simulink model "valve_02_sim"  (R2017b)
settings: Solver=VariableStepAuto  StartTime=0.0  StopTime=5  RelTol=1e-3
values from neighbouring files (symbols this model uses):
  fluid = nh3_v4    [valve_02.m]
undefined symbols (not defined in the file or in its folder): cp, cv, P, rho, T, Valve_regime, valveLib
libraries: simulink x4, thermochemical x4
settings Model: Creator=fferrucc  LastModifiedBy=fferrucc

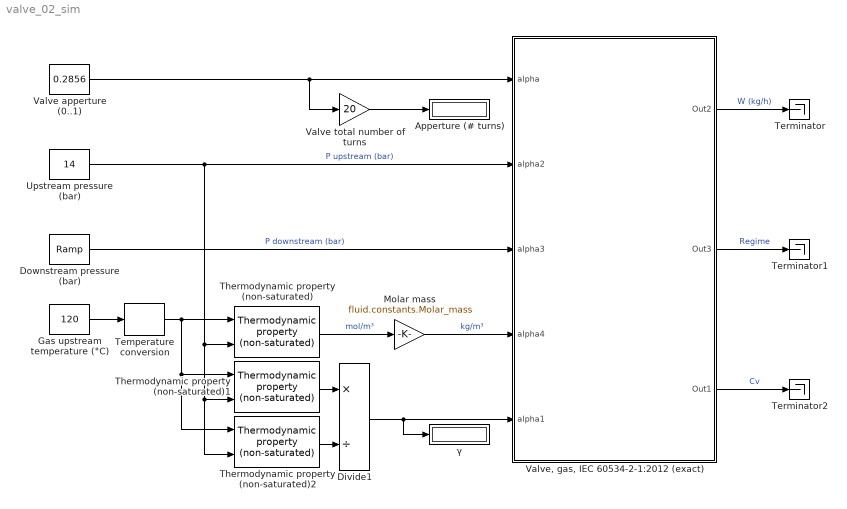
== system valve_02_sim ==
  Apperture (# turns) : Display
  Divide1 : Product  Inputs=*/
  "Downstream pressure (bar) " : simulink/Sources/Ramp  slope=1  start=0  X0=6
  Gas upstream temperature (°C) : Constant  Value=120
  Molar mass : Gain  Gain=fluid.constants.Molar_mass
  Temperature conversion : thermochemical/Conversions/Temperature conversion  sel=°C --> K
      settings: SourceProductName=@ Thermochemical
  Terminator : Terminator
  Terminator1 : Terminator
  Terminator2 : Terminator
  Thermodynamic property (non-saturated) : thermochemical/Thermodynamic fluid properties/Thermodynamic  property (non-saturated)  sel=rho(T,P)  fluid=fluid  reciprocVar=-1  lookup2D_BreakPoint1=fluid.no_sat.T_P_indep.var_indep.T  lookup2D_BreakPoint2=fluid.no_sat.T_P_indep.var_indep.P  lookup2D_Data=fluid.no_sat.T_P_indep.var_dep.rho_molar
      settings: SourceProductName=@ Thermochemical
  Thermodynamic property (non-saturated)1 : thermochemical/Thermodynamic fluid properties/Thermodynamic  property (non-saturated)  sel=cp(T,P)  fluid=fluid  reciprocVar=-1  lookup2D_BreakPoint1=fluid.no_sat.T_P_indep.var_indep.T  lookup2D_BreakPoint2=fluid.no_sat.T_P_indep.var_indep.P  lookup2D_Data=fluid.no_sat.T_P_indep.var_dep.Cp_molar
      settings: SourceProductName=@ Thermochemical
  Thermodynamic property (non-saturated)2 : thermochemical/Thermodynamic fluid properties/Thermodynamic  property (non-saturated)  sel=cv(T,P)  fluid=fluid  reciprocVar=-1  lookup2D_BreakPoint1=fluid.no_sat.T_P_indep.var_indep.T  lookup2D_BreakPoint2=fluid.no_sat.T_P_indep.var_indep.P  lookup2D_Data=fluid.no_sat.T_P_indep.var_dep.Cv_molar
      settings: SourceProductName=@ Thermochemical
  Upstream pressure (bar) : Constant  Value=14
  Valve apperture (0..1) : Constant  Value=0.2856
  Valve total number of turns : Gain  Gain=20
  "Valve, gas, IEC 60534-2-1:2012 (exact)" : Subsystem  AncestorBlock=thermochemical/Valves/Valve, gas, IEC 60534-2-1:2012 (exact)  mask(valve_gas_IEC60534_2_1_exact){Cv_dataPoints=valveLib.Hoke.s2300.model_2335G4Y.Cv_vs_apperture(:,2), apperture_dataPoints=valveLib.Hoke.s2300.model_2335G4Y.Cv_vs_apperture(:,1), xT=0.5}
      mask prompts: Cv_dataPoints "Cv vs apperture: Cv data points [0..Cv max]"; apperture_dataPoints "Cv vs apperture: apperture data points [0..1]"; xT "Pressure difference ratio factor of valve without attached fittings at choked flow ('xT' parameter) (use 0.5 if unknown)"
      mask help:
      | Model of a gas flow rate through a valve.
      |
      | The model takes into account the subcritical (non-chocked) and supercritical (chocked) regime of the pressure drop in the valve, switching its behaviour accordingly.
      |
      | The valve apperture is modulated by the signal 'apperture' (apperture = [0..1]).
      |
      | The model expects a table with the values of Cv (flow coeficient) as a function of the valve apperture (0..1).
      | NOTE: the relationship between Cv (imperial units) and Kv (SI units) is: Kv = 0.865*Cv.
      |
      | All the numerical outputs of the model are eigher positive or zero.
      mask DialogControl Control3 Prompt: Visit SWAGELOK site for more information about valves.
      mask DialogControl Control3 Callback: web('https://www.swagelok.com/en/Resources/CVCalculator','-browser')
  γ : Display
  wires:
  "Valve, gas, IEC 60534-2-1:2012 (exact)"/3(Out1) -> Terminator2/1  "Cv"
  "Valve, gas, IEC 60534-2-1:2012 (exact)"/2(Out3) -> Terminator1/1  "Regime"
  "Valve, gas, IEC 60534-2-1:2012 (exact)"/1(Out2) -> Terminator/1  "W (kg/h)"
  Thermodynamic property (non-saturated)/1 -> Molar mass/1  "mol/m³"
  Thermodynamic property (non-saturated)2/1 -> Divide1/2
  Thermodynamic property (non-saturated)1/1 -> Divide1/1
  Molar mass/1 -> "Valve, gas, IEC 60534-2-1:2012 (exact)"/4(alpha4)  "kg/m³"
  Upstream pressure (bar)/1 -> "Valve, gas, IEC 60534-2-1:2012 (exact)"/2(alpha2), Thermodynamic property (non-saturated)/2, Thermodynamic property (non-saturated)2/2, Thermodynamic property (non-saturated)1/2  "P upstream (bar)"
  Gas upstream temperature (°C)/1 -> Temperature conversion/1
  Divide1/1 -> γ/1, "Valve, gas, IEC 60534-2-1:2012 (exact)"/5(alpha1)
  Temperature conversion/1 -> Thermodynamic property (non-saturated)/1, Thermodynamic property (non-saturated)2/1, Thermodynamic property (non-saturated)1/1
  Valve apperture (0..1)/1 -> "Valve, gas, IEC 60534-2-1:2012 (exact)"/1(alpha), Valve total number of turns/1
  Valve total number of turns/1 -> Apperture (# turns)/1
  "Downstream pressure (bar) "/1 -> "Valve, gas, IEC 60534-2-1:2012 (exact)"/3(alpha3)  "P downstream (bar)"

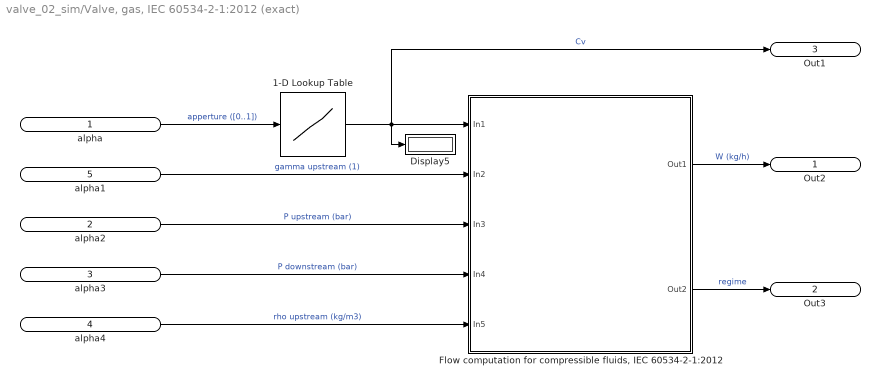
== system valve_02_sim/Valve, gas, IEC 60534-2-1:2012 (exact) ==
  alpha : Inport
  alpha2 : Inport  Port=2
  alpha3 : Inport  Port=3
  alpha4 : Inport  Port=4
  alpha1 : Inport  Port=5
  1-D Lookup Table : Lookup_n-D  NumberOfTableDimensions=1  BreakpointsForDimension1=apperture_dataPoints  BeginIndexSearchUsingPreviousIndexResult=on  Table=Cv_dataPoints  ExtrapMethod=Clip  InternalRulePriority=Speed  RndMeth=Simplest  InputSameDT=on
  Display5 : Display
  "Flow computation for compressible fluids, IEC 60534-2-1:2012" : Subsystem  LoadFcn=|
      | % For the 'regime' output to work, the model defines an enumerated type:
      | Simulink.defineIntEnumType('Valve_regime',{'Open_NonChocked','Closed','Open_Chocked'},[1 0 -1])
  Out2 : Outport
  Out3 : Outport  Port=2
  Out1 : Outport  Port=3
  wires:
  alpha4/1 -> "Flow computation for compressible fluids, IEC 60534-2-1:2012"/5(In5)  "rho upstream (kg/m3)"
  alpha3/1 -> "Flow computation for compressible fluids, IEC 60534-2-1:2012"/4(In4)  "P downstream (bar)"
  alpha2/1 -> "Flow computation for compressible fluids, IEC 60534-2-1:2012"/3(In3)  "P upstream (bar)"
  alpha1/1 -> "Flow computation for compressible fluids, IEC 60534-2-1:2012"/2(In2)  "gamma upstream (1)"
  1-D Lookup Table/1 -> "Flow computation for compressible fluids, IEC 60534-2-1:2012"/1(In1), Display5/1, Out1/1  "Cv"
  "Flow computation for compressible fluids, IEC 60534-2-1:2012"/2(Out2) -> Out3/1  "regime"
  alpha/1 -> 1-D Lookup Table/1  "apperture ([0..1])"
  "Flow computation for compressible fluids, IEC 60534-2-1:2012"/1(Out1) -> Out2/1  "W (kg/h)"

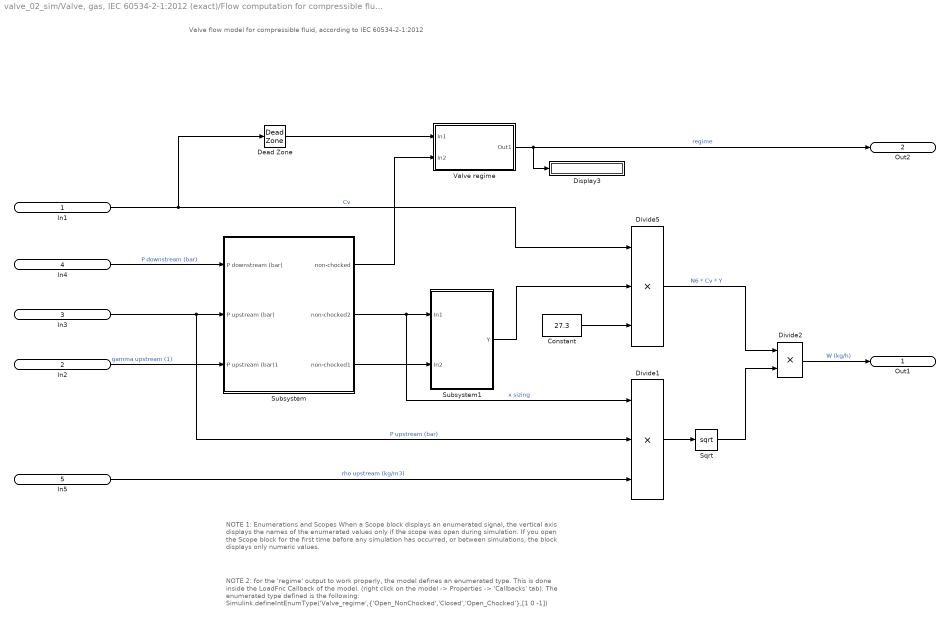
== system valve_02_sim/Valve, gas, IEC 60534-2-1:2012 (exact)/Flow computation for compressible fluids, IEC 60534-2-1:2012 ==
  note: NOTE 1: Enumerations and Scopes
      | When a Scope block displays an enumerated signal, the vertical axis displays the names of
      | the enumerated values only if the scope was open during simulation. If you open the Scope
      | block for the first time before any simulation has occurred, or between simulations, the block
      | displays only numeric values.
  note: NOTE 2: for the 'regime' output to work properly, the model defines an enumerated type. This is done
      | inside the LoadFnc Callback of the model. (right click on the model -> Properties -> 'Callbacks' tab).
      | The enumerated type defined is the following:
      | Simulink.defineIntEnumType('Valve_regime',{'Open_NonChocked','Closed','Open_Chocked'},[1 0 -1])
  note: Valve flow model for compressible fluid,
      | according to IEC 60534-2-1:2012
  In1 : Inport
  In2 : Inport  Port=2
  In3 : Inport  Port=3
  In4 : Inport  Port=4
  In5 : Inport  Port=5
  Constant : Constant  Value=27.3
  Dead Zone : DeadZone  LowerValue=-Inf  UpperValue=1e-7  SaturateOnIntegerOverflow=on
  Display3 : Display
  Divide1 : Product  Inputs=***
  Divide2 : Product  Inputs=**
  Divide5 : Product  Inputs=***
  Sqrt : Sqrt  SaturateOnIntegerOverflow=on
  Subsystem : Subsystem
  Subsystem1 : Subsystem
  Valve regime : Subsystem
  Out1 : Outport
  Out2 : Outport  Port=2
  wires:
  Dead Zone/1 -> Valve regime/1(In1)
  Valve regime/1(Out1) -> Display3/1, Out2/1  "regime"
  In4/1 -> Subsystem/1(P downstream (bar))  "P downstream (bar)"
  In3/1 -> Divide1/2, Subsystem/2(P upstream (bar))  "P upstream (bar)"
  In2/1 -> Subsystem/3(P upstream (bar)1)  "gamma upstream (1)"
  Subsystem/2(non-chocked2) -> Subsystem1/1(In1), Divide1/1  "x sizing"
  Subsystem/3(non-chocked1) -> Subsystem1/2(In2)
  In1/1 -> Dead Zone/1, Divide5/1  "Cv"
  Subsystem1/1(Y) -> Divide5/2
  Constant/1 -> Divide5/3
  Divide5/1 -> Divide2/1  "N6 * Cv * Y"
  In5/1 -> Divide1/3  "rho upstream (kg/m3)"
  Divide1/1 -> Sqrt/1
  Sqrt/1 -> Divide2/2
  Divide2/1 -> Out1/1  "W (kg/h)"
  Subsystem/1(non-chocked) -> Valve regime/2(In2)

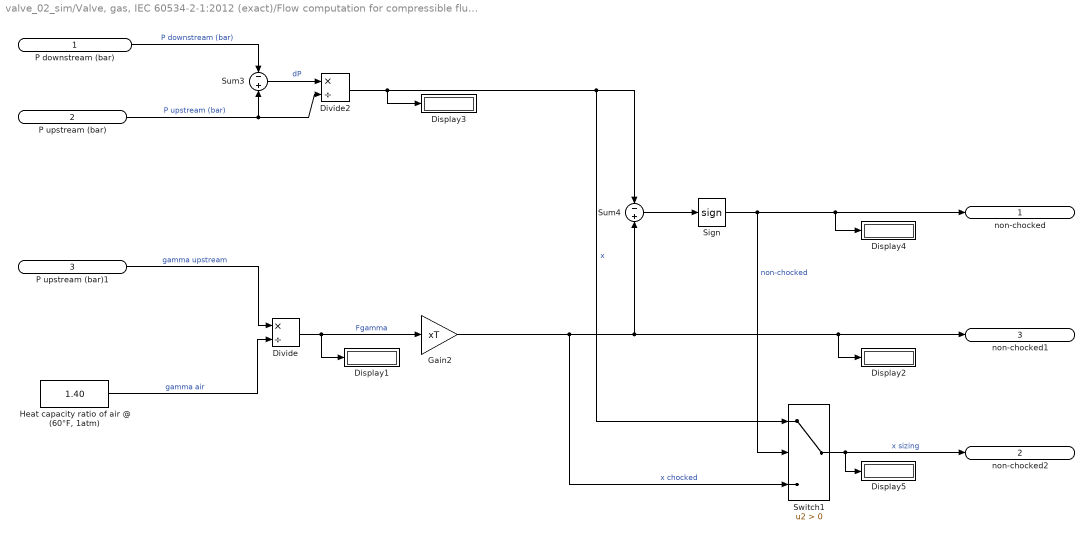
== system valve_02_sim/Valve, gas, IEC 60534-2-1:2012 (exact)/Flow computation for compressible fluids, IEC 60534-2-1:2012/Subsystem ==
  P downstream (bar) : Inport
  P upstream (bar) : Inport  Port=2
  P upstream (bar)1 : Inport  Port=3
  Display{1..5} (5 alike) : Display
  Divide : Product  Inputs=*/
  Divide2 : Product  Inputs=*/
  Gain2 : Gain  Gain=xT
  "Heat capacity ratio of air @ (60°F, 1atm)" : Constant  Value=1.40
  Sign : Signum
  Sum3 : Sum  Inputs=-+
  Sum4 : Sum  Inputs=-+
  Switch1 : Switch  Criteria=u2 > Threshold
  non-chocked : Outport
  non-chocked2 : Outport  Port=2
  non-chocked1 : Outport  Port=3
  wires:
  Divide/1 -> Gain2/1, Display1/1  "Fgamma"
  "Heat capacity ratio of air @ (60°F, 1atm)"/1 -> Divide/2  "gamma air"
  P upstream (bar)1/1 -> Divide/1  "gamma upstream"
  Divide2/1 -> Switch1/1, Sum4/1, Display3/1  "x"
  Sum3/1 -> Divide2/1  "dP"
  Sum4/1 -> Sign/1
  Gain2/1 -> Sum4/2, non-chocked1/1, Display2/1, Switch1/3  "x chocked"
  Sign/1 -> non-chocked/1, Display4/1, Switch1/2  "non-chocked"
  P downstream (bar)/1 -> Sum3/1  "P downstream (bar)"
  P upstream (bar)/1 -> Sum3/2, Divide2/2  "P upstream (bar)"
  Switch1/1 -> non-chocked2/1, Display5/1  "x sizing"

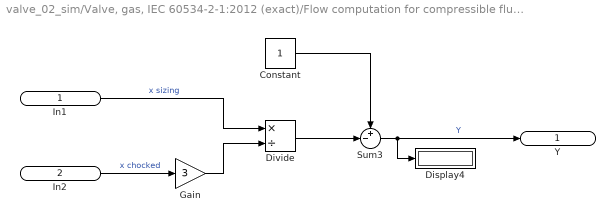
== system valve_02_sim/Valve, gas, IEC 60534-2-1:2012 (exact)/Flow computation for compressible fluids, IEC 60534-2-1:2012/Subsystem1 ==
  In1 : Inport
  In2 : Inport  Port=2
  Constant : Constant
  Display4 : Display
  Divide : Product  Inputs=*/
  Gain : Gain  Gain=3
  Sum3 : Sum  Inputs=+-|
  Y : Outport
  wires:
  Constant/1 -> Sum3/1
  In1/1 -> Divide/1  "x sizing"
  Gain/1 -> Divide/2
  Sum3/1 -> Y/1, Display4/1  "Y"
  In2/1 -> Gain/1  "x chocked"
  Divide/1 -> Sum3/2

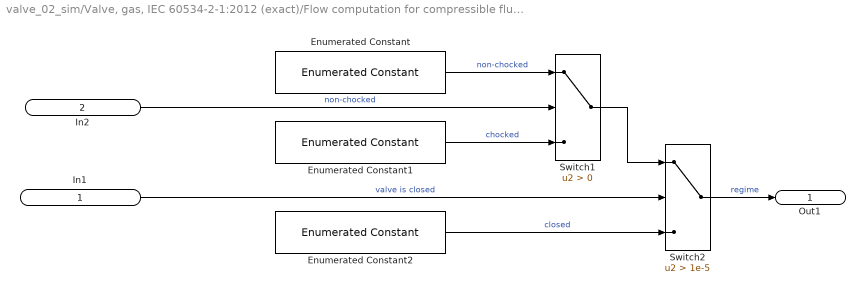
== system valve_02_sim/Valve, gas, IEC 60534-2-1:2012 (exact)/Flow computation for compressible fluids, IEC 60534-2-1:2012/Valve regime ==
  In1 : Inport
  In2 : Inport  Port=2
  Enumerated Constant : simulink/Sources/Enumerated Constant  OutDataTypeStr=Enum: Valve_regime  Value=Valve_regime.Open_NonChocked  SampleTime=inf
      settings: SourceProductName=Simulink
  Enumerated Constant1 : simulink/Sources/Enumerated Constant  OutDataTypeStr=Enum: Valve_regime  Value=Valve_regime.Open_Chocked  SampleTime=inf
      settings: SourceProductName=Simulink
  Enumerated Constant2 : simulink/Sources/Enumerated Constant  OutDataTypeStr=Enum: Valve_regime  Value=Valve_regime.Closed  SampleTime=inf
      settings: SourceProductName=Simulink
  Switch1 : Switch  Criteria=u2 > Threshold
  Switch2 : Switch  Criteria=u2 > Threshold  Threshold=1e-5
  Out1 : Outport
  wires:
  Switch1/1 -> Switch2/1
  Enumerated Constant/1 -> Switch1/1  "non-chocked"
  Enumerated Constant1/1 -> Switch1/3  "chocked"
  Enumerated Constant2/1 -> Switch2/3  "closed"
  Switch2/1 -> Out1/1  "regime"
  In2/1 -> Switch1/2  "non-chocked"
  In1/1 -> Switch2/2  "valve is closed"
